simulink model "transfer02"  (Simulink 7.7)
settings: Solver=ode45  StartTime=0.0  StopTime=10.0  MaxStep=.05  RelTol=1e-3
values from neighbouring files (symbols this model uses):
  B = 10    [setupPID.m]
  D = 100    [setupPID.m]
  J = m*L^2    (= 9)    [setupInvPend.m]    (also in setupPID.m = 0.1)
  Kd = 1749    [setupInvPend.m]    (also in setupPID.m = 2.56637061436)
  Ki = 0    [setupInvPend.m]    (also in setupPID.m = 4961.00426885)
  Kp = 85000    [setupInvPend.m]    (also in setupPID.m = 394.784176044)
libraries: simulink x2
settings Model: Creator=Rob  LastModifiedBy=rjwood
settings OptimizationCC: InitFltsAndDblsToZero=on
settings DebuggingCC: SaveWithParameterizedLinksMsg=none  SignalResolutionControl=TryResolveAllWithWarning  StrictBusMsg=Warning
settings GRTTargetCC: TargetFcnLib=ansi_tfl_tmw.mat

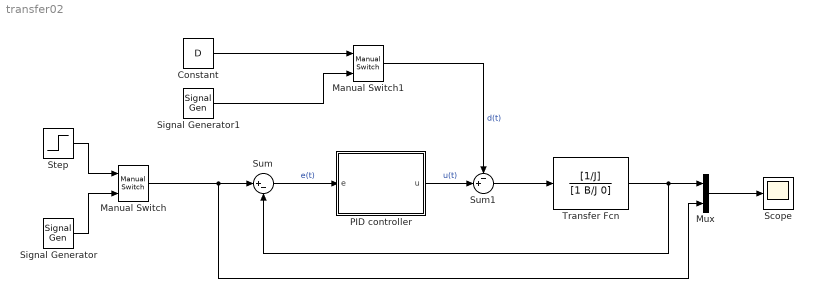
== system transfer02 ==
  Constant : Constant  Value=D
  Manual Switch : simulink/Signal Routing/Manual Switch  SystemSampleTime=-1  sw=0  action=0  varsize=off
  Manual Switch1 : simulink/Signal Routing/Manual Switch  SystemSampleTime=-1  sw=1  action=0  varsize=off
  Mux : Mux  Inputs=2
  PID controller : Subsystem
  Scope : Scope
  Signal Generator : SignalGenerator  WaveForm=sawtooth  Frequency=10
  Signal Generator1 : SignalGenerator  Amplitude=D  Frequency=0.33
  Step : Step  SampleTime=0
  Sum : Sum  Inputs=|+-
  Sum1 : Sum  Inputs=-+|
  Transfer Fcn : TransferFcn  Numerator=[1/J]  Denominator=[1 B/J 0]
  wires:
  Transfer Fcn/1 -> Mux/1, Sum/2
  Mux/1 -> Scope/1
  Sum/1 -> PID controller/1(e)  "e(t)"
  Manual Switch/1 -> Mux/2, Sum/1
  Step/1 -> Manual Switch/1
  Signal Generator/1 -> Manual Switch/2
  PID controller/1(u) -> Sum1/2  "u(t)"
  Sum1/1 -> Transfer Fcn/1
  Constant/1 -> Manual Switch1/1
  Manual Switch1/1 -> Sum1/1  "d(t)"
  Signal Generator1/1 -> Manual Switch1/2

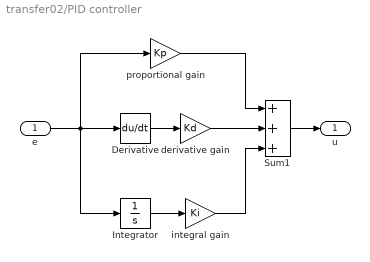
== system transfer02/PID controller ==
  e : Inport
  Derivative : Derivative
  Integrator : Integrator
  Sum1 : Sum  Inputs=+++
  derivative gain : Gain  Gain=Kd
  integral gain : Gain  Gain=Ki
  proportional gain : Gain  Gain=Kp
  u : Outport
  wires:
  e/1 -> proportional gain/1, Derivative/1, Integrator/1
  Derivative/1 -> derivative gain/1
  proportional gain/1 -> Sum1/1
  derivative gain/1 -> Sum1/2
  Sum1/1 -> u/1
  Integrator/1 -> integral gain/1
  integral gain/1 -> Sum1/3
